simulink model "Mdl_Dim"  (R2024b)
settings: Solver=FixedStepDiscrete  StartTime=0.0  StopTime=10.0  FixedStep=0.1  RelTol=1e-3  EnableMultiTasking=on
values from neighbouring files (symbols this model uses):
  DEFAULT_MODE = mpt.Parameter    [Mdl_Dim_DD.m]
  DEFAULT_STEP = mpt.Parameter    [Mdl_Dim_DD.m]
  Mdl_Dim_cTaskPeriod = mpt.Parameter    [Mdl_Dim_rte_types.m]
  RTE_E_MAX_AGE_EXCEEDED = mpt.Parameter    [Mdl_Dim_rte_types.m]
  RTE_E_NEVER_RECEIVED = mpt.Parameter    [Mdl_Dim_rte_types.m]
  STATUS_OFF = mpt.Parameter    [Mdl_Dim_DD.m]
  STATUS_ON = mpt.Parameter    [Mdl_Dim_DD.m]
  SWITCHING_MECHANISM = mpt.Parameter    [Mdl_Dim_DD.m]
  ZERO_VAL = mpt.Parameter    [Mdl_Dim_DD.m]
undefined symbols (not defined in the file or in its folder): AppModule, CAN_COMUN_ACTIVE, CAN_COMUN_FAIL, CAN_VAL_OFF, CAN_VAL_ON, ChannelID, CLUSTER_ACTIVE, DAYNIGHT_STS_NOTRequire, DIAG_NCTRL, DIM_DAY_MODE, DIM_NIGHT_MODE, DOWN_THRESH_1SW, DrvRec_Rheo_down_Long_Press, DrvRec_Rheo_down_Short_Press, DrvRec_Rheo_up_Long_Press, DrvRec_Rheo_Up_Short_Press, DW_EVENT, DW_ON, eAppMdl_type_instance, eDayNightModeIn, eIllumination_levelIn, eSIGNAL_MISSING, eSIGNAL_NEVER_RECEIVED, eSleepSt_type_instance, FALSE, GetPwmDirect, GetPwmWithTime, GetPwmWithTimeExp, IgnOn, INDEX_MCUID0340, INDEX_MCUID0341, INDEX_MCUID0430, IoHwAb_PwmSignalIdType_type_instance, l_Wheel_Down_ParamArray, l_Wheel_Up_ParamArray, MAX_UINT16, MAXHOLD, MINHOLD, NETWORK_NORMAL, NETWORK_SLEEP, NETWORK_STANDALONE, NONE, NVM_Adapter_SetNVM_RheostatDayStep, NVM_Adapter_SetNVM_RheostatDayStepU1, NVM_Adapter_SetNVM_RheostatDayStepU2, NVM_Adapter_SetNVM_RheostatDayStepU3, NVM_Adapter_SetNVM_RheostatNightStep, NVM_Adapter_SetNVM_RheostatNightStepU1, NVM_Adapter_SetNVM_RheostatNightStepU2, NVM_Adapter_SetNVM_RheostatNightStepU3, OpeModeRheostatChange, pJustRcvdStatus, pNvmData, POS_MAX, POS_MIN, RHEO_1SW_TYPE, RHEO_2SW_TYPE, RHEO_SOFTSW_TYPE, RHEO_VALUE_FIVE_U16, RHEO_VALUE_ONE_BOOL ... (+48)
libraries: simulink x65
(part 2 of 4)

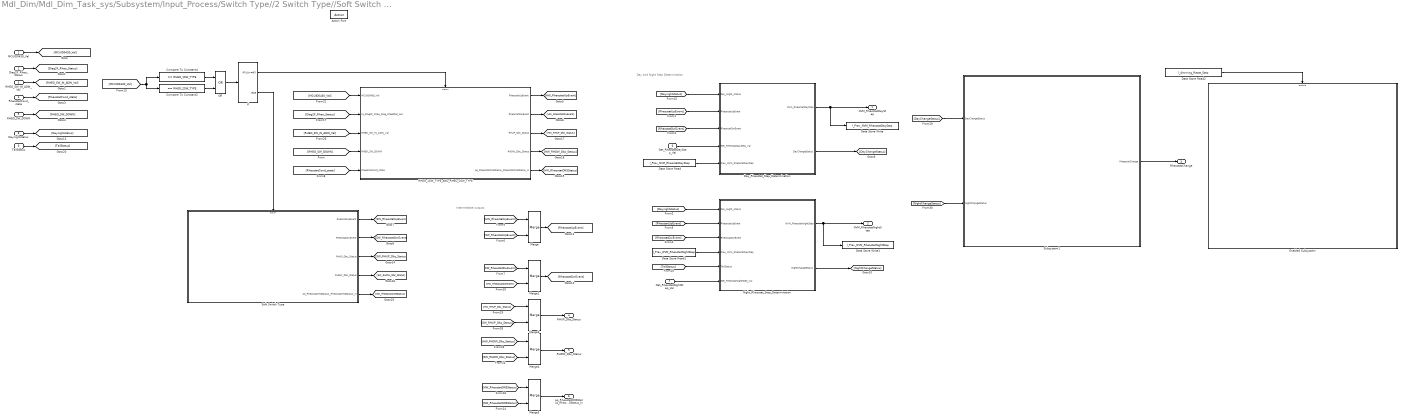
== system Mdl_Dim/Mdl_Dim_Task_sys/Subsystem/Input_Process/Switch Type//2 Switch Type//Soft Switch Type ==
  note: Intermediate outputs
  note: Day and Night Step Determination
  MCUID0430_Val : Inport
  Diag2F_Rheo_Status : Inport  Port=2
  RHEO_SW_IN_ADIN_Val : Inport  Port=3
  RheostatCond_state : Inport  Port=4
  RHEO_SW_DOWN : Inport  Port=5
  Get_RheostatDayStep_Val : Inport  Port=6
  Get_RheostatNightStep_Val : Inport  Port=7
  Daynightstatus : Inport  Port=8
  TailStatus : Inport  Port=9
  Action Port : ActionPort
  Compare To Constant2 : simulink/Logic and Bit Operations/Compare To Constant  relop===  const=RHEO_2SW_TYPE  OutDataTypeStr=boolean
  Compare To Constant4 : simulink/Logic and Bit Operations/Compare To Constant  relop===  const=RHEO_1SW_TYPE  OutDataTypeStr=boolean
  Data Store Read : DataStoreRead  DataStoreName=l_Prev_NVM_RheostatDayStep  IndexOptions=Index vector (dialog)  Indices=1  OutputSizes=1
  Data Store Read1 : DataStoreRead  DataStoreName=l_Prev_NVM_RheostatNightStep  IndexOptions=Index vector (dialog)  Indices=1  OutputSizes=1
  Data Store Read2 : DataStoreRead  DataStoreName=l_dimming_Reset_Step  IndexOptions=Index vector (dialog)  Indices=1  OutputSizes=1
  Data Store Write : DataStoreWrite  DataStoreName=l_Prev_NVM_RheostatDayStep  IndexOptions=Index vector (dialog)  Indices=1  OutputSizes=1
  Data Store Write1 : DataStoreWrite  DataStoreName=l_Prev_NVM_RheostatNightStep  IndexOptions=Index vector (dialog)  Indices=1  OutputSizes=1
  Day_Rheostat_Step_Determination : Truth Table  Priority=2  TreatAsAtomicUnit=on
      settings: RTWSystemCode=Nonreusable function  RTWFcnNameOpts=Use subsystem name
  Enabled Subsystem : Subsystem  Priority=3  TreatAsAtomicUnit=on
  If : If  IfExpression=(u1~=0)
  Merge{,1,3..5} (5 alike) : Merge
  Night_Rheostat_Step_Determination : Truth Table  Priority=2  TreatAsAtomicUnit=on
      settings: RTWSystemCode=Nonreusable function  RTWFcnNameOpts=Use subsystem name
  OR : Logic  Operator=OR  AllPortsSameDT=off  OutDataTypeStr=boolean
  RHEO_1SW_TYPE_AND_RHEO_2SW_TYPE : Subsystem  RTWFcnName=ONE_TWO_SWITCH_HANDLING
      settings: RTWSystemCode=Nonreusable function  RTWFcnNameOpts=User specified
  Soft Switch Type : Subsystem  RTWFcnName=SOFT_SWITCH_HANDLING
      settings: RTWSystemCode=Nonreusable function  RTWFcnNameOpts=User specified
  Subsystem1 : Subsystem  Priority=2
  "NVM_RheostatDayStep " : Outport  VectorParamsAs1DForOutWhenUnconnected=off
  NVM_RheostatNightStep : Outport  Port=2  VectorParamsAs1DForOutWhenUnconnected=off
  RheostatChange : Outport  Port=3  VectorParamsAs1DForOutWhenUnconnected=off
  RHUP_Dbc_Status : Outport  Port=4  VectorParamsAs1DForOutWhenUnconnected=off
  RHDW_Dbc_Status : Outport  Port=5  VectorParamsAs1DForOutWhenUnconnected=off
  pp_RheostatONSStatus_RheostatONSStatus_In : Outport  Port=6  VectorParamsAs1DForOutWhenUnconnected=off
  wires:
  [MCUID0430_Val] -> Compare To Constant4/1, Compare To Constant2/1
  [RheostatCond_state] -> RHEO_1SW_TYPE_AND_RHEO_2SW_TYPE/5(RheostatCond_state)
  [RHEO_SW_IN_ADIN_Val] -> RHEO_1SW_TYPE_AND_RHEO_2SW_TYPE/3(RHEO_SW_IN_ADIN_Val)
  [Diag2F_Rheo_Status] -> RHEO_1SW_TYPE_AND_RHEO_2SW_TYPE/2(rp_Diag2F_Rheo_Diag_RheoStat_out)
  [MCUID0430_Val] -> RHEO_1SW_TYPE_AND_RHEO_2SW_TYPE/1(MCUID0430_Val)
  Compare To Constant4/1 -> OR/1
  Compare To Constant2/1 -> OR/2
  MCUID0430_Val/1 -> [MCUID0430_Val]
  Diag2F_Rheo_Status/1 -> [Diag2F_Rheo_Status]
  RHEO_SW_IN_ADIN_Val/1 -> [RHEO_SW_IN_ADIN_Val]
  RheostatCond_state/1 -> [RheostatCond_state]
  RHEO_SW_DOWN/1 -> [RHEO_SW_DOWN]
  [RHEO_SW_DOWN] -> RHEO_1SW_TYPE_AND_RHEO_2SW_TYPE/4(RHEO_SW_DOWN)
  OR/1 -> If/1
  If/1 -> RHEO_1SW_TYPE_AND_RHEO_2SW_TYPE/Action
  If/2 -> Soft Switch Type/Action
  RHEO_1SW_TYPE_AND_RHEO_2SW_TYPE/1(RheostatUpEvent) -> [HW_RheostatUpEvent]
  RHEO_1SW_TYPE_AND_RHEO_2SW_TYPE/2(RheostatDwEvent) -> [HW_RheostatDwEvent]
  Soft Switch Type/1(RheostatUpEvent) -> [SW_RheostatUpEvent]
  Soft Switch Type/2(RheostatDwEvent) -> [SW_RheostatDwEvent]
  [HW_RheostatUpEvent] -> Merge/1
  [SW_RheostatUpEvent] -> Merge/2
  [SW_RheostatDwEvent] -> Merge1/1
  [HW_RheostatDwEvent] -> Merge1/2
  Merge/1 -> [RheostatUpEvent]
  Merge1/1 -> [RheostatDwEvent]
  [RheostatUpEvent] -> Day_Rheostat_Step_Determination/2(RheostatUpEvent)
  [RheostatDwEvent] -> Day_Rheostat_Step_Determination/3(RheostatDwEvent)
  Get_RheostatDayStep_Val/1 -> Day_Rheostat_Step_Determination/4(Get_RheostatDayStep_Val)
  [Daynightstatus] -> Day_Rheostat_Step_Determination/1(Day_Night_status)
  Day_Rheostat_Step_Determination/2(DayChangeStatus) -> [DayChangeStatus]
  Day_Rheostat_Step_Determination/1(NVM_RheostatDayStep) -> Data Store Write/1, "NVM_RheostatDayStep "/1
  Data Store Read/1 -> Day_Rheostat_Step_Determination/5(Prev_NVM_RheostatDayStep)
  Data Store Read1/1 -> Night_Rheostat_Step_Determination/4(Prev_NVM_RheostatDayStep)
  [TailStatus] -> Night_Rheostat_Step_Determination/5(TailStatus)
  [Daynightstatus] -> Night_Rheostat_Step_Determination/1(Day_Night_status)
  Night_Rheostat_Step_Determination/2(NightChangeStatus) -> [NightChangeStatus]
  [RheostatDwEvent] -> Night_Rheostat_Step_Determination/3(RheostatDwEvent)
  [RheostatUpEvent] -> Night_Rheostat_Step_Determination/2(RheostatUpEvent)
  Night_Rheostat_Step_Determination/1(NVM_RheostatNightStep) -> Data Store Write1/1, NVM_RheostatNightStep/1
  Get_RheostatNightStep_Val/1 -> Night_Rheostat_Step_Determination/6(Get_RheostatNightStep_Val)
  Daynightstatus/1 -> [Daynightstatus]
  Merge5/1 -> pp_RheostatONSStatus_RheostatONSStatus_In/1
  Soft Switch Type/3(RHUP_Dbc_Status) -> [SW_RHUP_Dbc_Status]
  Soft Switch Type/4(RHDW_Dbc_Status) -> [SW_RHDW_Dbc_Status]
  RHEO_1SW_TYPE_AND_RHEO_2SW_TYPE/3(RHUP_Dbc_Status) -> [HW_RHUP_Dbc_Status]
  RHEO_1SW_TYPE_AND_RHEO_2SW_TYPE/4(RHDW_Dbc_Status) -> [HW_RHDW_Dbc_Status]
  [HW_RHUP_Dbc_Status] -> Merge3/1
  [SW_RHUP_Dbc_Status] -> Merge3/2
  Merge3/1 -> RHUP_Dbc_Status/1
  [HW_RHDW_Dbc_Status] -> Merge4/1
  [SW_RHDW_Dbc_Status] -> Merge4/2
  Merge4/1 -> RHDW_Dbc_Status/1
  RHEO_1SW_TYPE_AND_RHEO_2SW_TYPE/5(pp_RheostatONSStatus_RheostatONSStatus_In) -> [HW_RheostatONSStatus]
  [SW_RheostatONSStatus] -> Merge5/2
  [HW_RheostatONSStatus] -> Merge5/1
  Soft Switch Type/5(pp_RheostatONSStatus_RheostatONSStatus_In) -> [SW_RheostatONSStatus]
  TailStatus/1 -> [TailStatus]
  Subsystem1/1(RheostatChange) -> RheostatChange/1
  [NightChangeStatus] -> Subsystem1/2(NightChangeStatus)
  [DayChangeStatus] -> Subsystem1/1(DayChangeStatus)
  Data Store Read2/1 -> Enabled Subsystem/Enable

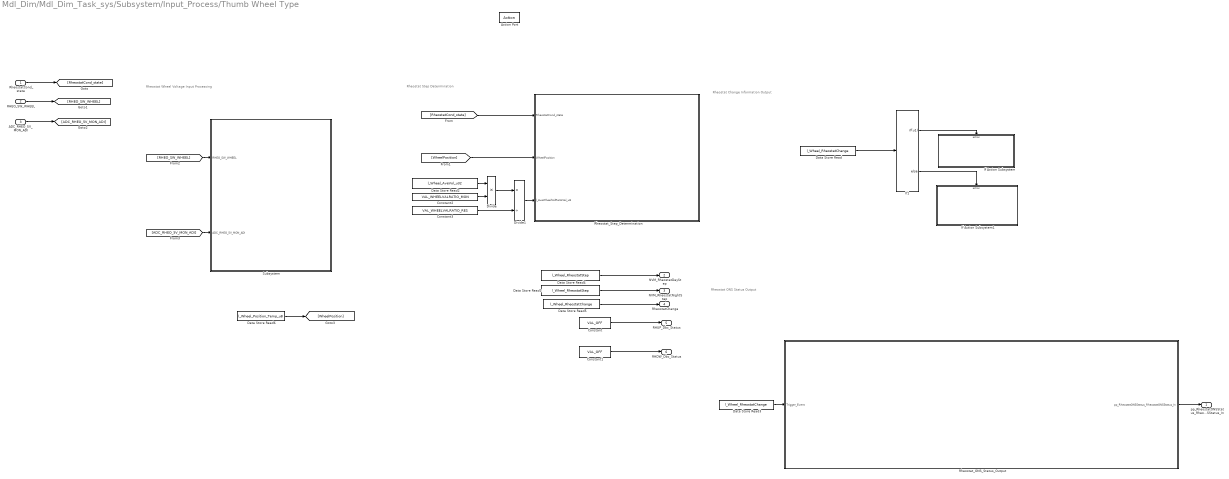
== system Mdl_Dim/Mdl_Dim_Task_sys/Subsystem/Input_Process/Thumb Wheel Type ==
  note: Rheostat Wheel Voltage Input Processing
  note: Rheostat Step Determination
  note: Rheostat Change Information Output
  note: Rheostat ONS Status Output
  RheostatCond_state : Inport
  RHEO_SW_WHEEL : Inport  Port=2
  ADC_RHEO_5V_MON_ADI : Inport  Port=3
  Action Port : ActionPort
  Constant : Constant  Value=VAL_OFF
  Constant1 : Constant  Value=VAL_OFF
  Constant2 : Constant  Value=VAL_WHEELVALRATIO_MON
  Constant3 : Constant  Value=VAL_WHEELVALRATIO_RES
  Data Store Read : DataStoreRead  DataStoreName=l_Wheel_RheostatChange  IndexOptions=Index vector (dialog)  Indices=1  OutputSizes=1
  Data Store Read1 : DataStoreRead  DataStoreName=l_Wheel_RheostatStep  IndexOptions=Index vector (dialog)  Indices=1  OutputSizes=1
  Data Store Read2 : DataStoreRead  DataStoreName=l_Wheel_AveVol_u32  IndexOptions=Index vector (dialog)  Indices=1  OutputSizes=1
  Data Store Read3 : DataStoreRead  DataStoreName=l_Wheel_RheostatChange  IndexOptions=Index vector (dialog)  Indices=1  OutputSizes=1
  Data Store Read4 : DataStoreRead  DataStoreName=l_Wheel_RheostatStep  IndexOptions=Index vector (dialog)  Indices=1  OutputSizes=1
  Data Store Read5 : DataStoreRead  DataStoreName=l_Wheel_RheostatChange  IndexOptions=Index vector (dialog)  Indices=1  OutputSizes=1
  Data Store Read6 : DataStoreRead  DataStoreName=l_Wheel_Position_Temp_u8  IndexOptions=Index vector (dialog)  Indices=1  OutputSizes=1
  Divide : Product  OutDataTypeStr=uint32
  Divide1 : Product  Inputs=*/  OutDataTypeStr=uint8
  If Action Subsystem : Subsystem  TreatAsAtomicUnit=on
  If Action Subsystem1 : Subsystem  TreatAsAtomicUnit=on
  If1 : If  IfExpression=u1
  "Rheostat_ONS_Status_Output " : Subsystem
  Rheostat_Step_Determination : Truth Table  TreatAsAtomicUnit=on
      settings: RTWSystemCode=Nonreusable function  RTWFcnNameOpts=Use subsystem name
  Subsystem : Subsystem
  pp_RheostatONSStatus_RheostatONSStatus_In : Outport  VectorParamsAs1DForOutWhenUnconnected=off
  "NVM_RheostatDayStep " : Outport  Port=2  VectorParamsAs1DForOutWhenUnconnected=off
  NVM_RheostatNightStep : Outport  Port=3  VectorParamsAs1DForOutWhenUnconnected=off
  RheostatChange : Outport  Port=4  VectorParamsAs1DForOutWhenUnconnected=off
  RHUP_Dbc_Status : Outport  Port=5  VectorParamsAs1DForOutWhenUnconnected=off
  RHDW_Dbc_Status : Outport  Port=6  VectorParamsAs1DForOutWhenUnconnected=off
  wires:
  "Rheostat_ONS_Status_Output "/1(pp_RheostatONSStatus_RheostatONSStatus_In) -> pp_RheostatONSStatus_RheostatONSStatus_In/1
  If1/2 -> If Action Subsystem1/Action
  If1/1 -> If Action Subsystem/Action
  Data Store Read/1 -> If1/1
  RHEO_SW_WHEEL/1 -> [RHEO_SW_WHEEL]
  ADC_RHEO_5V_MON_ADI/1 -> [ADC_RHEO_5V_MON_ADI]
  RheostatCond_state/1 -> [RheostatCond_state]
  [RheostatCond_state] -> Rheostat_Step_Determination/1(RheostatCond_state)
  Data Store Read5/1 -> RheostatChange/1
  Constant/1 -> RHUP_Dbc_Status/1
  Constant1/1 -> RHDW_Dbc_Status/1
  [WheelPosition] -> Rheostat_Step_Determination/2(WheelPosition)
  [RHEO_SW_WHEEL] -> Subsystem/1(RHEO_SW_WHEEL)
  [ADC_RHEO_5V_MON_ADI] -> Subsystem/2(ADC_RHEO_5V_MON_ADI)
  Data Store Read6/1 -> [WheelPosition]
  Data Store Read3/1 -> "Rheostat_ONS_Status_Output "/1(Trigger_Event)
  Data Store Read4/1 -> "NVM_RheostatDayStep "/1
  Data Store Read1/1 -> NVM_RheostatNightStep/1
  Constant3/1 -> Divide1/2
  Divide/1 -> Divide1/1
  Data Store Read2/1 -> Divide/1
  Constant2/1 -> Divide/2
  Divide1/1 -> Rheostat_Step_Determination/3(l_AveWheelVolRaitoVal_u8)

== system Mdl_Dim/Mdl_Dim_Task_sys/Subsystem/Input_Process/Switch Type//2 Switch Type//Soft Switch Type/Enabled Subsystem ==
  Enable : EnablePort
  Constant : Constant  Value=VAL_OFF
  Constant1 : Constant  Value=MAXHOLD
  Data Store Read : DataStoreRead  DataStoreName=l_Dim_MCUID0340_val  IndexOptions=Index vector (dialog)  Indices=1  OutputSizes=1
  Data Store Write : DataStoreWrite  DataStoreName=l_Prev_NVM_RheostatDayStep  IndexOptions=Index vector (dialog)  Indices=1  OutputSizes=1
  Data Store Write1 : DataStoreWrite  DataStoreName=l_Prev_NVM_RheostatNightStep  IndexOptions=Index vector (dialog)  Indices=1  OutputSizes=1
  Data Store Write2 : DataStoreWrite  DataStoreName=l_dimming_Reset_Step  IndexOptions=Index vector (dialog)  Indices=1  OutputSizes=1
  NVM_Adapter_SetNVM_RheostatDayStep : FunctionCaller  FunctionPrototype=NVM_Adapter_SetNVM_RheostatDayStep(pNvmData)  InputArgumentSpecifications=uint8(1)  OutputArgumentSpecifications=<Enter example>
  NVM_Adapter_SetNVM_RheostatDayStepU1 : FunctionCaller  FunctionPrototype=NVM_Adapter_SetNVM_RheostatDayStepU1(pNvmData)  InputArgumentSpecifications=uint8(1)  OutputArgumentSpecifications=<Enter example>
  NVM_Adapter_SetNVM_RheostatDayStepU2 : FunctionCaller  FunctionPrototype=NVM_Adapter_SetNVM_RheostatDayStepU2(pNvmData)  InputArgumentSpecifications=uint8(1)  OutputArgumentSpecifications=<Enter example>
  NVM_Adapter_SetNVM_RheostatDayStepU3 : FunctionCaller  FunctionPrototype=NVM_Adapter_SetNVM_RheostatDayStepU3(pNvmData)  InputArgumentSpecifications=uint8(1)  OutputArgumentSpecifications=<Enter example>
  NVM_Adapter_SetNVM_RheostatNightStep : FunctionCaller  FunctionPrototype=NVM_Adapter_SetNVM_RheostatNightStep(pNvmData)  InputArgumentSpecifications=uint8(1)  OutputArgumentSpecifications=<Enter example>
  NVM_Adapter_SetNVM_RheostatNightStep2 : FunctionCaller  FunctionPrototype=NVM_Adapter_SetNVM_RheostatNightStepU2(pNvmData)  InputArgumentSpecifications=uint8(1)  OutputArgumentSpecifications=<Enter example>
  NVM_Adapter_SetNVM_RheostatNightStepU1 : FunctionCaller  FunctionPrototype=NVM_Adapter_SetNVM_RheostatNightStepU1(pNvmData)  InputArgumentSpecifications=uint8(1)  OutputArgumentSpecifications=<Enter example>
  NVM_Adapter_SetNVM_RheostatNightStepU3 : FunctionCaller  FunctionPrototype=NVM_Adapter_SetNVM_RheostatNightStepU3(pNvmData)  InputArgumentSpecifications=uint8(1)  OutputArgumentSpecifications=<Enter example>
  wires:
  Constant/1 -> Data Store Write2/1
  Constant1/1 -> Data Store Write/1, NVM_Adapter_SetNVM_RheostatDayStep/1, NVM_Adapter_SetNVM_RheostatDayStepU3/1, NVM_Adapter_SetNVM_RheostatDayStepU2/1, NVM_Adapter_SetNVM_RheostatDayStepU1/1
  Data Store Read/1 -> NVM_Adapter_SetNVM_RheostatNightStep2/1, Data Store Write1/1, NVM_Adapter_SetNVM_RheostatNightStep/1, NVM_Adapter_SetNVM_RheostatNightStepU3/1, NVM_Adapter_SetNVM_RheostatNightStepU1/1

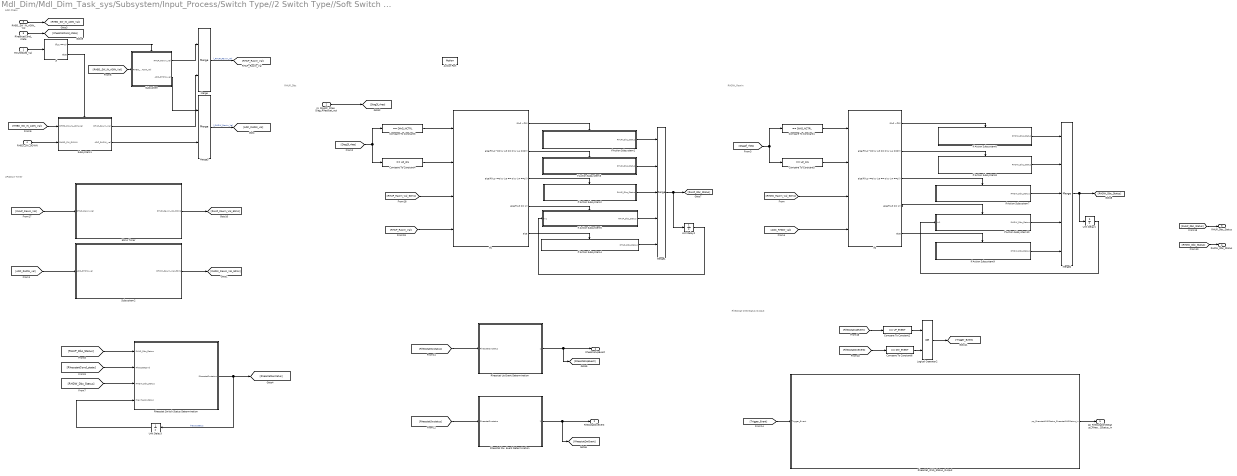
== system Mdl_Dim/Mdl_Dim_Task_sys/Subsystem/Input_Process/Switch Type//2 Switch Type//Soft Switch Type/RHEO_1SW_TYPE_AND_RHEO_2SW_TYPE ==
  note: Rheostat ONS Status Output
  note: RHDW_RawIn
  note: RHUP_Dbc
  note: UP/Down Timer
  note: ADC Check
  MCUID0430_Val : Inport
  rp_Diag2F_Rheo_Diag_RheoStat_out : Inport  Port=2
  RHEO_SW_IN_ADIN_Val : Inport  Port=3
  RHEO_SW_DOWN : Inport  Port=4
  RheostatCond_state : Inport  Port=5
  Action Port : ActionPort
  " Rheostat Dw  Event Determination" : Subsystem
  " Rheostat Up Event Determination" : Subsystem
  50ms Timer : Subsystem  Priority=1
      settings: AttributesFormatString=Priority = %<Priority>
  Compare To Constant1 : simulink/Logic and Bit Operations/Compare To Constant  relop===  const=DIAG_NCTRL  OutDataTypeStr=boolean
  Compare To Constant2 : simulink/Logic and Bit Operations/Compare To Constant  relop===  const=UP_EVENT  OutDataTypeStr=boolean
  Compare To Constant3 : simulink/Logic and Bit Operations/Compare To Constant  relop===  const=DIAG_NCTRL  OutDataTypeStr=boolean
  Compare To Constant4 : simulink/Logic and Bit Operations/Compare To Constant  relop===  const=UP_ON  OutDataTypeStr=boolean
  Compare To Constant5 : simulink/Logic and Bit Operations/Compare To Constant  relop===  const=UP_ON  OutDataTypeStr=boolean
  Compare To Constant6 : simulink/Logic and Bit Operations/Compare To Constant  relop===  const=DW_EVENT  OutDataTypeStr=boolean
  If : If  IfExpression=u1 == 0
  If Action Subsystem1 : Subsystem  TreatAsAtomicUnit=on
  If Action Subsystem10 : Subsystem  TreatAsAtomicUnit=on
  If Action Subsystem2 : Subsystem  TreatAsAtomicUnit=on
  If Action Subsystem3 : Subsystem  TreatAsAtomicUnit=on
  If Action Subsystem4 : Subsystem  TreatAsAtomicUnit=on
  If Action Subsystem5 : Subsystem  TreatAsAtomicUnit=on
  If Action Subsystem6 : Subsystem  TreatAsAtomicUnit=on
  If Action Subsystem7 : Subsystem  TreatAsAtomicUnit=on
  If Action Subsystem8 : Subsystem  TreatAsAtomicUnit=on
  If Action Subsystem9 : Subsystem  TreatAsAtomicUnit=on
  If1 : If  Priority=3  NumInputs=4  IfExpression=u2 ~=0  ElseIfExpressions=((u1~=0) & (u3 == 0) & (u4 ==0)) , ((u1~=0) & (u3 == 0) & (u4 ==1)),(u3 == 1)
      settings: AttributesFormatString=Priority = %<Priority>
  If2 : If  NumInputs=4  IfExpression=u2 ~=0  ElseIfExpressions=((u1~=0) & (u3 == 0) & (u4 ==0)) , ((u1~=0) & (u3 == 0) & (u4 ==1)),(u3 == 1)
  Logical Operator2 : Logic  Operator=OR  AllPortsSameDT=off  OutDataTypeStr=boolean
  Merge : Merge
  Merge1 : Merge  Inputs=5
  Merge2 : Merge  Inputs=5
  Merge3 : Merge
  Rheostat Switch Status Determination : Truth Table
  "Rheostat_ONS_Status_Output " : Subsystem
  Subsystem : Subsystem
  Subsystem1 : Subsystem
  Subsystem2 : Subsystem  Priority=2
      settings: AttributesFormatString=Priority = %<Priority>
  Unit Delay1 : UnitDelay  SampleTime=-1  StateName=l_Prev_SW1RHDW_Dbc_status  HasFrameUpgradeWarning=on
  Unit Delay2 : UnitDelay  SampleTime=-1  StateName=l_Prev_SW1RHUP_Dbc_status  HasFrameUpgradeWarning=on
  Unit Delay3 : UnitDelay  InitialCondition=UNKNOWNSTATUS  SampleTime=-1  StateName=l_Prev_RheostatswStatus  HasFrameUpgradeWarning=on
  RheostatUpEvent : Outport  VectorParamsAs1DForOutWhenUnconnected=off
  RheostatDwEvent : Outport  Port=2  VectorParamsAs1DForOutWhenUnconnected=off
  RHUP_Dbc_Status : Outport  Port=3  VectorParamsAs1DForOutWhenUnconnected=off
  RHDW_Dbc_Status : Outport  Port=4  VectorParamsAs1DForOutWhenUnconnected=off
  pp_RheostatONSStatus_RheostatONSStatus_In : Outport  Port=5  VectorParamsAs1DForOutWhenUnconnected=off
  wires:
  If1/3 -> If Action Subsystem2/Action
  Merge1/1 -> [RHUP_Dbc_Status], Unit Delay2/1
  Unit Delay2/1 -> If Action Subsystem5/1(In1)
  50ms Timer/1(RHUP_RawIn_Val_50ms) -> [RHUP_RawIn_Val_50ms]
  If Action Subsystem5/1(RHUP_Dbc_Status) -> Merge1/4
  Compare To Constant3/1 -> If1/1
  If1/2 -> If Action Subsystem3/Action
  If Action Subsystem4/1(RHUP_Dbc_Status) -> Merge1/5
  If1/4 -> If Action Subsystem5/Action
  [RHUP_RawIn_Val] -> If1/4
  If1/5 -> If Action Subsystem4/Action
  If Action Subsystem2/1(RHUP_Dbc_Status) -> Merge1/3
  If Action Subsystem1/1(RHUP_Dbc_Status) -> Merge1/1
  Compare To Constant4/1 -> If1/2
  [RHUP_RawIn_Val_50ms] -> If1/3
  [RHUP_RawIn_Val] -> 50ms Timer/1(RHUP_RawIn_Val)
  If1/1 -> If Action Subsystem1/Action
  If Action Subsystem3/1(RHUP_Dbc_Status) -> Merge1/2
  [Diag2f_rheo] -> Compare To Constant1/1, Compare To Constant5/1
  If2/1 -> If Action Subsystem6/Action
  If Action Subsystem8/1(RHDW_Dbc_Status) -> Merge2/2
  If Action Subsystem6/1(RHDW_Dbc_Status) -> Merge2/1
  If Action Subsystem7/1(RHDW_Dbc_Status) -> Merge2/3
  [RHDW_RawIn_Val_50ms] -> If2/3
  Compare To Constant5/1 -> If2/2
  [ADC_RHDW_val] -> If2/4
  If2/5 -> If Action Subsystem9/Action
  If2/4 -> If Action Subsystem10/Action
  If Action Subsystem9/1(RHDW_Dbc_Status) -> Merge2/5
  If2/2 -> If Action Subsystem8/Action
  Compare To Constant1/1 -> If2/1
  Merge2/1 -> Unit Delay1/1, [RHDW_Dbc_Status]
  Unit Delay1/1 -> If Action Subsystem10/1(In1)
  If Action Subsystem10/1(RHDW_Dbc_Status) -> Merge2/4
  If2/3 -> If Action Subsystem7/Action
  Subsystem2/1(RHDW_RawIn_Val_50ms) -> [RHDW_RawIn_Val_50ms]
  [ADC_RHDW_val] -> Subsystem2/1(ADC_RHDW_val)
  rp_Diag2F_Rheo_Diag_RheoStat_out/1 -> [Diag2f_rheo]
  [Diag2f_rheo] -> Compare To Constant4/1, Compare To Constant3/1
  RHEO_SW_IN_ADIN_Val/1 -> [RHEO_SW_IN_ADIN_Val]
  [RHEO_SW_IN_ADIN_Val] -> Subsystem/1(RHEO_SW_IN_ADIN_Val)
  RHEO_SW_DOWN/1 -> Subsystem1/2(RHEO_SW_DOWN)
  [RHEO_SW_IN_ADIN_Val] -> Subsystem1/1(RHEO_SW_IN_ADIN_Val)
  MCUID0430_Val/1 -> If/1
  If/1 -> Subsystem/Action
  If/2 -> Subsystem1/Action
  Subsystem/1(RHUP_RawIn_Val) -> Merge/1
  Subsystem1/1(RHUP_RawIn_Val) -> Merge/2
  Subsystem/2(ADC_RHDW_val) -> Merge3/1
  Subsystem1/2(ADC_RHDW_val) -> Merge3/2
  Merge/1 -> [RHUP_RawIn_Val]  "l_RHUP_RawIn_Val"
  Merge3/1 -> [ADC_RHDW_val]  "l_RHDW_RawIn_Val"
  [RheostatCond_state] -> Rheostat Switch Status Determination/2(RheostatCond)
  [RHUP_Dbc_Status] -> Rheostat Switch Status Determination/1(RHUP_Dbc_Status)
  Unit Delay3/1 -> Rheostat Switch Status Determination/4(Prevrheoswstatus)
  Rheostat Switch Status Determination/1(RheostatSwstatus) -> Unit Delay3/1, [RheostatSwstatus]  "rheoswstatus"
  [RHDW_Dbc_Status] -> Rheostat Switch Status Determination/3(RHDW_Dbc_Status)
  [RheostatSwstatus] -> " Rheostat Dw  Event Determination"/1(RheostatSwstatus)
  " Rheostat Dw  Event Determination"/1(" ") -> [RheostatDwEvent], RheostatDwEvent/1
  [RheostatSwstatus] -> " Rheostat Up Event Determination"/1(RheostatSwstatus)
  " Rheostat Up Event Determination"/1(" ") -> [RheostatUpEvent], RheostatUpEvent/1
  RheostatCond_state/1 -> [RheostatCond_state]
  [RHDW_Dbc_Status] -> RHDW_Dbc_Status/1
  [RHUP_Dbc_Status] -> RHUP_Dbc_Status/1
  [RheostatUpEvent] -> Compare To Constant2/1
  [RheostatDwEvent] -> Compare To Constant6/1
  Compare To Constant2/1 -> Logical Operator2/1
  Compare To Constant6/1 -> Logical Operator2/2
  Logical Operator2/1 -> [Trigger_Event]
  "Rheostat_ONS_Status_Output "/1(pp_RheostatONSStatus_RheostatONSStatus_In) -> pp_RheostatONSStatus_RheostatONSStatus_In/1
  [Trigger_Event] -> "Rheostat_ONS_Status_Output "/1(Trigger_Event)

== system Mdl_Dim/Mdl_Dim_Task_sys/Subsystem/Input_Process/Switch Type//2 Switch Type//Soft Switch Type/Soft Switch Type ==
  Action Port : ActionPort
  Constant : Constant  Value=VAL_OFF
  Constant1 : Constant  Value=VAL_OFF
  Constant2 : Constant  Value=VAL_OFF
  Constant3 : Constant  Value=VAL_OFF  OutDataTypeStr=uint32
  Data Store Write : DataStoreWrite  DataStoreName=l_Prev_Rheo3secCount  IndexOptions=Index vector (dialog)  Indices=1  OutputSizes=1
  Event Check : Subsystem  Priority=1
      settings: AttributesFormatString=Priority = %<Priority>
  Event Clear : Subsystem  Priority=2
      settings: AttributesFormatString=Priority = %<Priority>
  RheostatUpEvent : Outport  VectorParamsAs1DForOutWhenUnconnected=off
  RheostatDwEvent : Outport  Port=2  VectorParamsAs1DForOutWhenUnconnected=off
  RHUP_Dbc_Status : Outport  Port=3  VectorParamsAs1DForOutWhenUnconnected=off
  RHDW_Dbc_Status : Outport  Port=4  VectorParamsAs1DForOutWhenUnconnected=off
  pp_RheostatONSStatus_RheostatONSStatus_In : Outport  Port=5  VectorParamsAs1DForOutWhenUnconnected=off
  wires:
  Event Check/1(RheostatUpEvent) -> RheostatUpEvent/1
  Event Check/2(RheostatDwEvent) -> RheostatDwEvent/1
  Constant/1 -> RHUP_Dbc_Status/1
  Constant1/1 -> RHDW_Dbc_Status/1
  Constant2/1 -> pp_RheostatONSStatus_RheostatONSStatus_In/1
  Constant3/1 -> Data Store Write/1

== system Mdl_Dim/Mdl_Dim_Task_sys/Subsystem/Input_Process/Switch Type//2 Switch Type//Soft Switch Type/Subsystem1 ==
  note: Change Judgement
  DayChangeStatus : Inport
  NightChangeStatus : Inport  Port=2
  If Action Subsystem : Subsystem  TreatAsAtomicUnit=on
  If Action Subsystem1 : Subsystem  TreatAsAtomicUnit=on
  If1 : If  IfExpression=u1
  Logical Operator : Logic  Operator=OR  AllPortsSameDT=off  OutDataTypeStr=boolean
  Merge2 : Merge
  RheostatChange : Outport  VectorParamsAs1DForOutWhenUnconnected=off
  wires:
  If1/1 -> If Action Subsystem/Action
  Logical Operator/1 -> If1/1
  Merge2/1 -> RheostatChange/1
  If Action Subsystem1/1(RheostatChange) -> Merge2/2
  If1/2 -> If Action Subsystem1/Action
  [NightChangeStatus] -> Logical Operator/2
  If Action Subsystem/1(RheostatChange) -> Merge2/1
  [DayChangeStatus] -> Logical Operator/1
  DayChangeStatus/1 -> [DayChangeStatus]
  NightChangeStatus/1 -> [NightChangeStatus]

== system Mdl_Dim/Mdl_Dim_Task_sys/Subsystem/Input_Process/Thumb Wheel Type/If Action Subsystem ==
  Action Port : ActionPort
  Data Store Read1 : DataStoreRead  DataStoreName=l_Wheel_RheostatStep  IndexOptions=Index vector (dialog)  Indices=1  OutputSizes=1
  Data Store Read4 : DataStoreRead  DataStoreName=l_Wheel_RheostatStep  IndexOptions=Index vector (dialog)  Indices=1  OutputSizes=1
  NVM_Adapter_SetNVM_RheostatDayStep : FunctionCaller  FunctionPrototype=NVM_Adapter_SetNVM_RheostatDayStep(pNvmData)  InputArgumentSpecifications=uint8(1)  OutputArgumentSpecifications=<Enter example>
  NVM_Adapter_SetNVM_RheostatNightStep : FunctionCaller  FunctionPrototype=NVM_Adapter_SetNVM_RheostatNightStep(pNvmData)  InputArgumentSpecifications=uint8(1)  OutputArgumentSpecifications=<Enter example>
  OpeModeRheostatChange : FunctionCaller  FunctionPrototype=OpeModeRheostatChange()  InputArgumentSpecifications=<Enter example>  OutputArgumentSpecifications=<Enter example>
  wires:
  Data Store Read1/1 -> NVM_Adapter_SetNVM_RheostatNightStep/1
  Data Store Read4/1 -> NVM_Adapter_SetNVM_RheostatDayStep/1

== system Mdl_Dim/Mdl_Dim_Task_sys/Subsystem/Input_Process/Thumb Wheel Type/If Action Subsystem1 ==
  Action Port : ActionPort

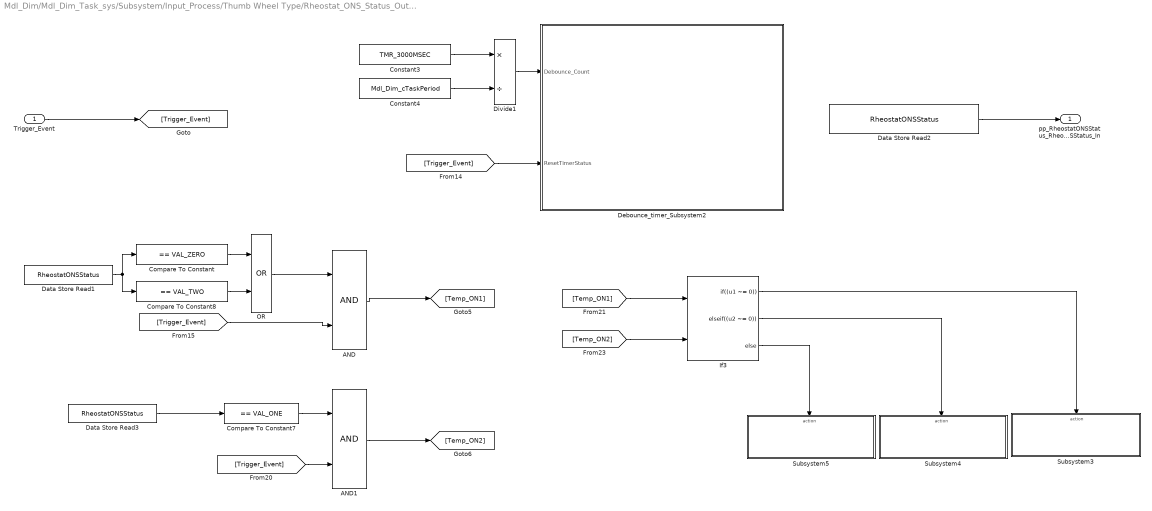
== system Mdl_Dim/Mdl_Dim_Task_sys/Subsystem/Input_Process/Thumb Wheel Type/Rheostat_ONS_Status_Output  ==
  Trigger_Event : Inport
  AND : Logic  AllPortsSameDT=off  OutDataTypeStr=boolean
  AND1 : Logic  AllPortsSameDT=off  OutDataTypeStr=boolean
  Compare To Constant : simulink/Logic and Bit Operations/Compare To Constant  relop===  const=VAL_ZERO  OutDataTypeStr=boolean
  Compare To Constant7 : simulink/Logic and Bit Operations/Compare To Constant  relop===  const=VAL_ONE  OutDataTypeStr=boolean
  Compare To Constant8 : simulink/Logic and Bit Operations/Compare To Constant  relop===  const=VAL_TWO  OutDataTypeStr=boolean
  Constant3 : Constant  Value=TMR_3000MSEC
  Constant4 : Constant  Value=Mdl_Dim_cTaskPeriod
  Data Store Read1 : DataStoreRead  DataStoreName=RheostatONSStatus  IndexOptions=Index vector (dialog)  Indices=1  OutputSizes=1
  Data Store Read2 : DataStoreRead  DataStoreName=RheostatONSStatus  IndexOptions=Index vector (dialog)  Indices=1  OutputSizes=1
  Data Store Read3 : DataStoreRead  DataStoreName=RheostatONSStatus  IndexOptions=Index vector (dialog)  Indices=1  OutputSizes=1
  Debounce_timer_Subsystem2 : Subsystem  Description=|
      | Input 1 : Deboune Count
      | Input 2 : Reset Timer Status
      | Output : Timer Debounce Status
  Divide1 : Product  Inputs=*/  OutDataTypeStr=uint16
  If3 : If  NumInputs=2  IfExpression=(u1 ~= 0)  ElseIfExpressions=(u2 ~= 0)
  OR : Logic  Operator=OR  AllPortsSameDT=off  OutDataTypeStr=boolean
  Subsystem3 : Subsystem
  Subsystem4 : Subsystem
  Subsystem5 : Subsystem
  pp_RheostatONSStatus_RheostatONSStatus_In : Outport  VectorParamsAs1DForOutWhenUnconnected=off
  wires:
  [Trigger_Event] -> AND1/2
  If3/3 -> Subsystem5/Action
  If3/2 -> Subsystem4/Action
  Constant3/1 -> Divide1/1
  Data Store Read1/1 -> Compare To Constant/1, Compare To Constant8/1
  Data Store Read3/1 -> Compare To Constant7/1
  [Temp_ON2] -> If3/2
  [Temp_ON1] -> If3/1
  AND1/1 -> [Temp_ON2]
  Data Store Read2/1 -> pp_RheostatONSStatus_RheostatONSStatus_In/1
  If3/1 -> Subsystem3/Action
  Compare To Constant/1 -> OR/1
  Compare To Constant7/1 -> AND1/1
  Compare To Constant8/1 -> OR/2
  Constant4/1 -> Divide1/2
  Divide1/1 -> Debounce_timer_Subsystem2/1(Debounce_Count)
  OR/1 -> AND/1
  [Trigger_Event] -> AND/2
  AND/1 -> [Temp_ON1]
  [Trigger_Event] -> Debounce_timer_Subsystem2/2("ResetTimerStatus ")
  Trigger_Event/1 -> [Trigger_Event]

== system Mdl_Dim/Mdl_Dim_Task_sys/Subsystem/Input_Process/Thumb Wheel Type/Subsystem ==
  RHEO_SW_WHEEL : Inport
  ADC_RHEO_5V_MON_ADI : Inport  Port=2
  Subsystem1 : Subsystem
  wires:
  RHEO_SW_WHEEL/1 -> [RHEO_SW_WHEEL]
  ADC_RHEO_5V_MON_ADI/1 -> [ADC_RHEO_5V_MON_ADI]
  [RHEO_SW_WHEEL] -> Subsystem1/1(RHEO_SW_WHEEL)
  [ADC_RHEO_5V_MON_ADI] -> Subsystem1/2(ADC_RHEO_5V_MON_ADI)

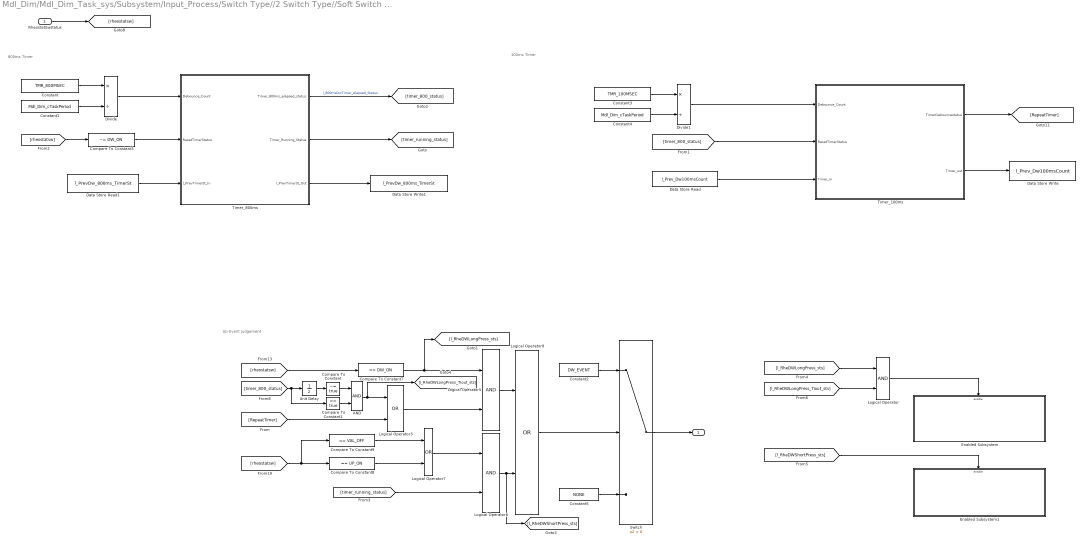
== system Mdl_Dim/Mdl_Dim_Task_sys/Subsystem/Input_Process/Switch Type//2 Switch Type//Soft Switch Type/RHEO_1SW_TYPE_AND_RHEO_2SW_TYPE/ Rheostat Dw  Event Determination ==
  note: 100ms Timer
  note: 800ms Timer
  note: Up Event judgement
  RheostatSwstatus : Inport
  AND : Logic  AllPortsSameDT=off  OutDataTypeStr=boolean
  Compare To Constant : simulink/Logic and Bit Operations/Compare To Constant  relop=~=  const=true  OutDataTypeStr=boolean
  Compare To Constant1 : simulink/Logic and Bit Operations/Compare To Constant  relop===  const=true  OutDataTypeStr=boolean
  Compare To Constant3 : simulink/Logic and Bit Operations/Compare To Constant  relop=~=  const=DW_ON  OutDataTypeStr=boolean
  Compare To Constant7 : simulink/Logic and Bit Operations/Compare To Constant  relop===  const=DW_ON  OutDataTypeStr=boolean
  Compare To Constant8 : simulink/Logic and Bit Operations/Compare To Constant  relop===  const=UP_ON  OutDataTypeStr=boolean
  Compare To Constant9 : simulink/Logic and Bit Operations/Compare To Constant  relop===  const=VAL_OFF  OutDataTypeStr=boolean
  Constant : Constant  Value=TMR_800MSEC
  Constant1 : Constant  Value=Mdl_Dim_cTaskPeriod
  Constant2 : Constant  Value=DW_EVENT
  Constant3 : Constant  Value=TMR_100MSEC
  Constant4 : Constant  Value=Mdl_Dim_cTaskPeriod
  Constant5 : Constant  Value=NONE
  Data Store Read : DataStoreRead  DataStoreName=l_Prev_Dw100msCount  IndexOptions=Index vector (dialog)  Indices=1  OutputSizes=1
  Data Store Read1 : DataStoreRead  DataStoreName=l_PrevDw_800ms_TimerSt  IndexOptions=Index vector (dialog)  Indices=1  OutputSizes=1
  Data Store Write : DataStoreWrite  DataStoreName=l_Prev_Dw100msCount  IndexOptions=Index vector (dialog)  Indices=1  OutputSizes=1
  Data Store Write1 : DataStoreWrite  DataStoreName=l_PrevDw_800ms_TimerSt  IndexOptions=Index vector (dialog)  Indices=1  OutputSizes=1
  Divide : Product  Inputs=*/  OutDataTypeStr=uint16
  Divide1 : Product  Inputs=*/  OutDataTypeStr=uint16
  Enabled Subsystem : Subsystem  TreatAsAtomicUnit=on
  Enabled Subsystem1 : Subsystem  TreatAsAtomicUnit=on
  Logical Operator : Logic  AllPortsSameDT=off  OutDataTypeStr=boolean
  Logical Operator3 : Logic  Operator=OR  AllPortsSameDT=off  OutDataTypeStr=boolean
  Logical Operator5 : Logic  AllPortsSameDT=off  OutDataTypeStr=boolean
  Logical Operator6 : Logic  AllPortsSameDT=off  OutDataTypeStr=boolean
  Logical Operator7 : Logic  Operator=OR  AllPortsSameDT=off  OutDataTypeStr=boolean
  Logical Operator8 : Logic  Operator=OR  AllPortsSameDT=off  OutDataTypeStr=boolean
  Switch : Switch  Criteria=u2 > Threshold  SaturateOnIntegerOverflow=off  InputSameDT=off
  Timer_100ms : Subsystem  Description=|  TreatAsAtomicUnit=on  RTWFcnName=Timer_100ms
      | Input 1 : Deboune Count
      | Input 2 : Reset Timer Status
      | Output : Timer Debounce Status
      settings: RTWFcnNameOpts=User specified
  Timer_800ms : Subsystem  Description=|  TreatAsAtomicUnit=on  RTWFcnName=Timer_800ms
      | Input 1 : Deboune Count
      | Input 2 : Reset Timer Status
      | Output : Timer Debounce Status
      settings: RTWFcnNameOpts=User specified
  Unit Delay : UnitDelay  SampleTime=-1  StateName=Prev_Dw_timer_800_status  HasFrameUpgradeWarning=on
  " " : Outport  VectorParamsAs1DForOutWhenUnconnected=off
  wires:
  Constant1/1 -> Divide/2
  Constant/1 -> Divide/1
  Timer_800ms/1(Timer_800ms_elapsed_status) -> [timer_800_status]  "l_800msDwTimer_elapsed_Status"
  Divide/1 -> Timer_800ms/1(Debounce_Count)
  Constant3/1 -> Divide1/1
  Constant4/1 -> Divide1/2
  RheostatSwstatus/1 -> [rheostatsw]
  [rheostatsw] -> Compare To Constant3/1
  Compare To Constant3/1 -> Timer_800ms/2("ResetTimerStatus ")
  Divide1/1 -> Timer_100ms/1(Debounce_Count)
  Timer_100ms/1(TimerDebouncestatus) -> [RepeatTimer]
  Timer_800ms/2(Timer_Running_Status) -> [timer_running_status]
  [timer_800_status] -> Timer_100ms/2("ResetTimerStatus ")
  Data Store Read1/1 -> Timer_800ms/3(l_PrevTimerSt_In)
  Timer_800ms/3(l_PrevTimerSt_Out) -> Data Store Write1/1
  Timer_100ms/2(Timer_out) -> Data Store Write/1
  Data Store Read/1 -> Timer_100ms/3(Timer_In)
  AND/1 -> [l_RheDWLongPress_Tiout_sts], Logical Operator3/1
  Compare To Constant9/1 -> Logical Operator7/1
  [rheostatsw] -> Compare To Constant7/1
  [rheostatsw] -> Compare To Constant8/1, Compare To Constant9/1
  [timer_running_status] -> Logical Operator6/2
  [l_RheDWLongPress_sts] -> Logical Operator/1
  Logical Operator7/1 -> Logical Operator6/1
  Switch/1 -> " "/1
  Compare To Constant8/1 -> Logical Operator7/2
  [l_RheDWLongPress_Tiout_sts] -> Logical Operator/2
  Compare To Constant/1 -> AND/1
  [timer_800_status] -> Compare To Constant1/1, Unit Delay/1
  Unit Delay/1 -> Compare To Constant/1
  Logical Operator8/1 -> Switch/2
  Compare To Constant7/1 -> [l_RheDWLongPress_sts], Logical Operator5/1
  Compare To Constant1/1 -> AND/2
  [RepeatTimer] -> Logical Operator3/2
  Logical Operator5/1 -> Logical Operator8/1
  Constant2/1 -> Switch/1
  Constant5/1 -> Switch/3
  Logical Operator3/1 -> Logical Operator5/2
  Logical Operator6/1 -> [l_RheDWShortPress_sts], Logical Operator8/2
  Logical Operator/1 -> Enabled Subsystem/Enable
  [l_RheDWShortPress_sts] -> Enabled Subsystem1/Enable

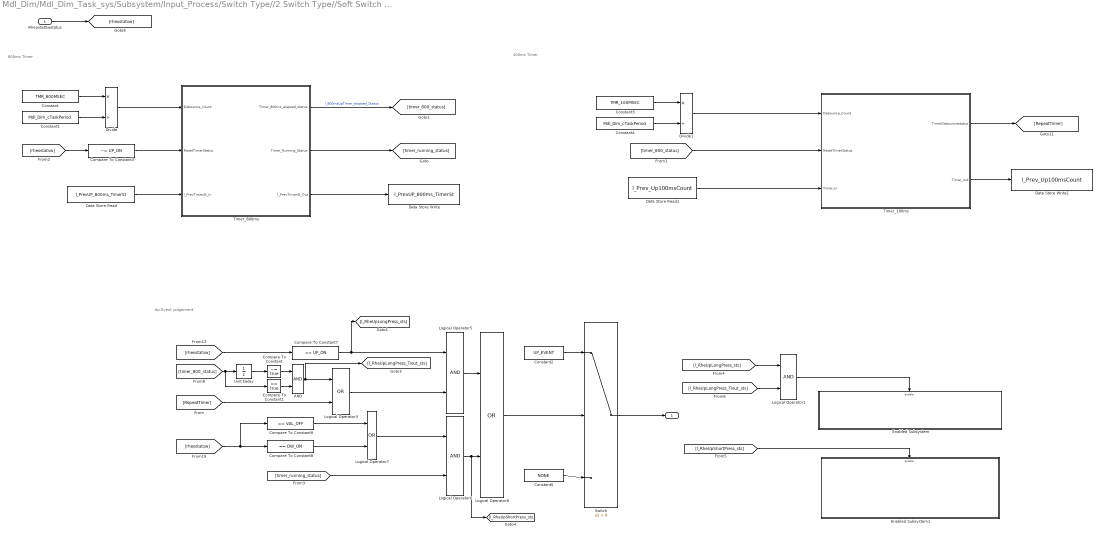
== system Mdl_Dim/Mdl_Dim_Task_sys/Subsystem/Input_Process/Switch Type//2 Switch Type//Soft Switch Type/RHEO_1SW_TYPE_AND_RHEO_2SW_TYPE/ Rheostat Up Event Determination ==
  note: 100ms Timer
  note: 800ms Timer
  note: Up Event judgement
  RheostatSwstatus : Inport
  AND : Logic  AllPortsSameDT=off  OutDataTypeStr=boolean
  Compare To Constant : simulink/Logic and Bit Operations/Compare To Constant  relop=~=  const=true  OutDataTypeStr=boolean
  Compare To Constant1 : simulink/Logic and Bit Operations/Compare To Constant  relop===  const=true  OutDataTypeStr=boolean
  Compare To Constant3 : simulink/Logic and Bit Operations/Compare To Constant  relop=~=  const=UP_ON  OutDataTypeStr=boolean
  Compare To Constant7 : simulink/Logic and Bit Operations/Compare To Constant  relop===  const=UP_ON  OutDataTypeStr=boolean
  Compare To Constant8 : simulink/Logic and Bit Operations/Compare To Constant  relop===  const=DW_ON  OutDataTypeStr=boolean
  Compare To Constant9 : simulink/Logic and Bit Operations/Compare To Constant  relop===  const=VAL_OFF  OutDataTypeStr=boolean
  Constant : Constant  Value=TMR_800MSEC
  Constant1 : Constant  Value=Mdl_Dim_cTaskPeriod
  Constant2 : Constant  Value=UP_EVENT
  Constant3 : Constant  Value=TMR_100MSEC
  Constant4 : Constant  Value=Mdl_Dim_cTaskPeriod
  Constant5 : Constant  Value=NONE
  Data Store Read : DataStoreRead  DataStoreName=l_PrevUP_800ms_TimerSt  IndexOptions=Index vector (dialog)  Indices=1  OutputSizes=1
  Data Store Read1 : DataStoreRead  DataStoreName=l_Prev_Up100msCount  IndexOptions=Index vector (dialog)  Indices=1  OutputSizes=1
  Data Store Write : DataStoreWrite  DataStoreName=l_PrevUP_800ms_TimerSt  IndexOptions=Index vector (dialog)  Indices=1  OutputSizes=1
  Data Store Write1 : DataStoreWrite  DataStoreName=l_Prev_Up100msCount  IndexOptions=Index vector (dialog)  Indices=1  OutputSizes=1
  Divide : Product  Inputs=*/  OutDataTypeStr=uint16
  Divide1 : Product  Inputs=*/  OutDataTypeStr=uint16
  Enabled Subsystem : Subsystem  TreatAsAtomicUnit=on
  Enabled Subsystem1 : Subsystem  TreatAsAtomicUnit=on
  Logical Operator1 : Logic  AllPortsSameDT=off  OutDataTypeStr=boolean
  Logical Operator3 : Logic  Operator=OR  AllPortsSameDT=off  OutDataTypeStr=boolean
  Logical Operator5 : Logic  AllPortsSameDT=off  OutDataTypeStr=boolean
  Logical Operator6 : Logic  AllPortsSameDT=off  OutDataTypeStr=boolean
  Logical Operator7 : Logic  Operator=OR  AllPortsSameDT=off  OutDataTypeStr=boolean
  Logical Operator8 : Logic  Operator=OR  AllPortsSameDT=off  OutDataTypeStr=boolean
  Switch : Switch  Criteria=u2 > Threshold  SaturateOnIntegerOverflow=off  InputSameDT=off
  Timer_100ms : Subsystem  Description=|  TreatAsAtomicUnit=on  RTWFcnName=Timer_100ms
      | Input 1 : Deboune Count
      | Input 2 : Reset Timer Status
      | Output : Timer Debounce Status
      settings: RTWFcnNameOpts=User specified
  Timer_800ms : Subsystem  Description=|  TreatAsAtomicUnit=on  RTWFcnName=Timer_800ms
      | Input 1 : Deboune Count
      | Input 2 : Reset Timer Status
      | Output : Timer Debounce Status
      settings: RTWFcnNameOpts=User specified
  Unit Delay : UnitDelay  SampleTime=-1  StateName=Prev_timer_800_status  HasFrameUpgradeWarning=on
  " " : Outport  VectorParamsAs1DForOutWhenUnconnected=off
  wires:
  Constant1/1 -> Divide/2
  Constant/1 -> Divide/1
  Timer_800ms/1(Timer_800ms_elapsed_status) -> [timer_800_status]  "l_800msUpTimer_elapsed_Status"
  Divide/1 -> Timer_800ms/1(Debounce_Count)
  Constant3/1 -> Divide1/1
  Constant4/1 -> Divide1/2
  RheostatSwstatus/1 -> [rheostatsw]
  [rheostatsw] -> Compare To Constant3/1
  Compare To Constant3/1 -> Timer_800ms/2("ResetTimerStatus ")
  Divide1/1 -> Timer_100ms/1(Debounce_Count)
  Timer_100ms/1(TimerDebouncestatus) -> [RepeatTimer]
  Timer_800ms/2(Timer_Running_Status) -> [timer_running_status]
  [timer_800_status] -> Timer_100ms/2("ResetTimerStatus ")
  Timer_800ms/3(l_PrevTimerSt_Out) -> Data Store Write/1
  Data Store Read/1 -> Timer_800ms/3(l_PrevTimerSt_In)
  Timer_100ms/2(Timer_out) -> Data Store Write1/1
  Data Store Read1/1 -> Timer_100ms/3(Timer_In)
  Switch/1 -> " "/1
  Logical Operator7/1 -> Logical Operator6/1
  [l_RheUpLongPress_Tiout_sts] -> Logical Operator1/2
  [l_RheUpLongPress_sts] -> Logical Operator1/1
  Unit Delay/1 -> Compare To Constant/1
  AND/1 -> [l_RheUpLongPress_Tiout_sts], Logical Operator3/1
  Logical Operator3/1 -> Logical Operator5/2
  [rheostatsw] -> Compare To Constant8/1, Compare To Constant9/1
  [timer_running_status] -> Logical Operator6/2
  Compare To Constant9/1 -> Logical Operator7/1
  [RepeatTimer] -> Logical Operator3/2
  [rheostatsw] -> Compare To Constant7/1
  Compare To Constant/1 -> AND/1
  Logical Operator5/1 -> Logical Operator8/1
  Logical Operator8/1 -> Switch/2
  Compare To Constant8/1 -> Logical Operator7/2
  Logical Operator6/1 -> [l_RheUpShortPress_sts], Logical Operator8/2
  Compare To Constant7/1 -> [l_RheUpLongPress_sts], Logical Operator5/1
  Compare To Constant1/1 -> AND/2
  Constant2/1 -> Switch/1
  [timer_800_status] -> Compare To Constant1/1, Unit Delay/1
  Constant5/1 -> Switch/3
  Logical Operator1/1 -> Enabled Subsystem/Enable
  [l_RheUpShortPress_sts] -> Enabled Subsystem1/Enable

== system Mdl_Dim/Mdl_Dim_Task_sys/Subsystem/Input_Process/Switch Type//2 Switch Type//Soft Switch Type/RHEO_1SW_TYPE_AND_RHEO_2SW_TYPE/50ms Timer ==
  RHUP_RawIn_Val : Inport
  AND : Logic  AllPortsSameDT=off  OutDataTypeStr=boolean
  Compare To Constant : simulink/Logic and Bit Operations/Compare To Constant  relop=~=  const=RHEO_VALUE_ZERO_BOOL  OutDataTypeStr=boolean
  Compare To Constant1 : simulink/Logic and Bit Operations/Compare To Constant  relop=~=  const=RHEO_VALUE_ONE_BOOL  OutDataTypeStr=boolean
  Compare To Constant5 : simulink/Logic and Bit Operations/Compare To Constant  relop===  const=RHEO_VALUE_ONE_BOOL  OutDataTypeStr=boolean
  Constant1 : Constant  Value=RHEO_VALUE_ZERO_U16  OutDataTypeStr=Inherit: Inherit via back propagation
  Constant4 : Constant  Value=RHEO_VALUE_ONE_U16  OutDataTypeStr=uint16
  Constant5 : Constant  Value=RHEO_VALUE_ZERO_U16  OutDataTypeStr=Inherit: Inherit via back propagation
  Constant7 : Constant  Value=RHEO_VALUE_FIVE_U16  OutDataTypeStr=uint16
  Subtract1 : Sum  Inputs=+-
  Switch2 : Switch  Criteria=u2 ~= 0  OutDataTypeStr=uint16  SaturateOnIntegerOverflow=off  InputSameDT=off
  Switch3 : Switch  Criteria=u2 ~= 0  OutDataTypeStr=uint16  RndMeth=Simplest  SaturateOnIntegerOverflow=off  InputSameDT=off
  Unit Delay : UnitDelay  SampleTime=-1  StateName=Prev_RHUP_RawIn_Val  HasFrameUpgradeWarning=on
  Unit Delay2 : UnitDelay  InitialCondition=ZERO_DUTY  SampleTime=-1  StateName=Prev_SW1Rheostat_Up_time_Step50ms  HasFrameUpgradeWarning=on
  check count2 : RelationalOperator  Operator=~=  OutDataTypeStr=boolean  InputSameDT=off
  RHUP_RawIn_Val_50ms : Outport  VectorParamsAs1DForOutWhenUnconnected=off
  wires:
  Unit Delay2/1 -> Switch2/3  "current_count_2"
  Switch2/1 -> Subtract1/1, check count2/1  "current_count_2"
  check count2/1 -> RHUP_RawIn_Val_50ms/1, Switch3/2  "fl_RHUP_RawIn_Val_50ms"
  Compare To Constant5/1 -> Switch2/2
  Constant4/1 -> Subtract1/2  "Decrement_Value_2"
  Constant7/1 -> Switch2/1  "Decrement_Value_2fRheo"
  Switch3/1 -> Unit Delay2/1
  Constant5/1 -> check count2/2  "Max_step_Count2"
  RHUP_RawIn_Val/1 -> [RHUP_RawIn_Val], Unit Delay/1
  Unit Delay/1 -> [Prev_RHUP_RawIn_Val]
  AND/1 -> Compare To Constant5/1
  Subtract1/1 -> Switch3/1  "current_count_2"
  Constant1/1 -> Switch3/3
  [RHUP_RawIn_Val] -> Compare To Constant/1
  Compare To Constant/1 -> AND/1
  Compare To Constant1/1 -> AND/2
  [Prev_RHUP_RawIn_Val] -> Compare To Constant1/1

== system Mdl_Dim/Mdl_Dim_Task_sys/Subsystem/Input_Process/Switch Type//2 Switch Type//Soft Switch Type/RHEO_1SW_TYPE_AND_RHEO_2SW_TYPE/If Action Subsystem1 ==
  Action Port : ActionPort
  Constant : Constant  Value=VAL_ON  OutDataTypeStr=uint8
  RHUP_Dbc_Status : Outport  VectorParamsAs1DForOutWhenUnconnected=off
  wires:
  Constant/1 -> RHUP_Dbc_Status/1

== system Mdl_Dim/Mdl_Dim_Task_sys/Subsystem/Input_Process/Switch Type//2 Switch Type//Soft Switch Type/RHEO_1SW_TYPE_AND_RHEO_2SW_TYPE/If Action Subsystem10 ==
  In1 : Inport
  Action Port : ActionPort
  RHDW_Dbc_Status : Outport  VectorParamsAs1DForOutWhenUnconnected=off
  wires:
  In1/1 -> RHDW_Dbc_Status/1

== system Mdl_Dim/Mdl_Dim_Task_sys/Subsystem/Input_Process/Switch Type//2 Switch Type//Soft Switch Type/RHEO_1SW_TYPE_AND_RHEO_2SW_TYPE/If Action Subsystem2 ==
  Action Port : ActionPort
  Constant : Constant  Value=VAL_ON  OutDataTypeStr=uint8
  RHUP_Dbc_Status : Outport  VectorParamsAs1DForOutWhenUnconnected=off
  wires:
  Constant/1 -> RHUP_Dbc_Status/1

== system Mdl_Dim/Mdl_Dim_Task_sys/Subsystem/Input_Process/Switch Type//2 Switch Type//Soft Switch Type/RHEO_1SW_TYPE_AND_RHEO_2SW_TYPE/If Action Subsystem3 ==
  Action Port : ActionPort
  Constant : Constant  Value=VAL_OFF  OutDataTypeStr=uint8
  RHUP_Dbc_Status : Outport  VectorParamsAs1DForOutWhenUnconnected=off
  wires:
  Constant/1 -> RHUP_Dbc_Status/1

== system Mdl_Dim/Mdl_Dim_Task_sys/Subsystem/Input_Process/Switch Type//2 Switch Type//Soft Switch Type/RHEO_1SW_TYPE_AND_RHEO_2SW_TYPE/If Action Subsystem4 ==
  Action Port : ActionPort
  Constant : Constant  Value=VAL_OFF  OutDataTypeStr=uint8
  RHUP_Dbc_Status : Outport  VectorParamsAs1DForOutWhenUnconnected=off
  wires:
  Constant/1 -> RHUP_Dbc_Status/1

== system Mdl_Dim/Mdl_Dim_Task_sys/Subsystem/Input_Process/Switch Type//2 Switch Type//Soft Switch Type/RHEO_1SW_TYPE_AND_RHEO_2SW_TYPE/If Action Subsystem5 ==
  In1 : Inport
  Action Port : ActionPort
  RHUP_Dbc_Status : Outport  VectorParamsAs1DForOutWhenUnconnected=off
  wires:
  In1/1 -> RHUP_Dbc_Status/1

== system Mdl_Dim/Mdl_Dim_Task_sys/Subsystem/Input_Process/Switch Type//2 Switch Type//Soft Switch Type/RHEO_1SW_TYPE_AND_RHEO_2SW_TYPE/If Action Subsystem6 ==
  Action Port : ActionPort
  Constant : Constant  Value=VAL_ON  OutDataTypeStr=uint8
  RHDW_Dbc_Status : Outport  VectorParamsAs1DForOutWhenUnconnected=off
  wires:
  Constant/1 -> RHDW_Dbc_Status/1

== system Mdl_Dim/Mdl_Dim_Task_sys/Subsystem/Input_Process/Switch Type//2 Switch Type//Soft Switch Type/RHEO_1SW_TYPE_AND_RHEO_2SW_TYPE/If Action Subsystem7 ==
  Action Port : ActionPort
  Constant : Constant  Value=VAL_ON  OutDataTypeStr=uint8
  RHDW_Dbc_Status : Outport  VectorParamsAs1DForOutWhenUnconnected=off
  wires:
  Constant/1 -> RHDW_Dbc_Status/1

== system Mdl_Dim/Mdl_Dim_Task_sys/Subsystem/Input_Process/Switch Type//2 Switch Type//Soft Switch Type/RHEO_1SW_TYPE_AND_RHEO_2SW_TYPE/If Action Subsystem8 ==
  Action Port : ActionPort
  Constant : Constant  Value=VAL_OFF  OutDataTypeStr=uint8
  RHDW_Dbc_Status : Outport  VectorParamsAs1DForOutWhenUnconnected=off
  wires:
  Constant/1 -> RHDW_Dbc_Status/1

== system Mdl_Dim/Mdl_Dim_Task_sys/Subsystem/Input_Process/Switch Type//2 Switch Type//Soft Switch Type/RHEO_1SW_TYPE_AND_RHEO_2SW_TYPE/If Action Subsystem9 ==
  Action Port : ActionPort
  Constant : Constant  Value=VAL_OFF  OutDataTypeStr=uint8
  RHDW_Dbc_Status : Outport  VectorParamsAs1DForOutWhenUnconnected=off
  wires:
  Constant/1 -> RHDW_Dbc_Status/1

== system Mdl_Dim/Mdl_Dim_Task_sys/Subsystem/Input_Process/Switch Type//2 Switch Type//Soft Switch Type/RHEO_1SW_TYPE_AND_RHEO_2SW_TYPE/Rheostat_ONS_Status_Output  ==
  Trigger_Event : Inport
  AND : Logic  AllPortsSameDT=off  OutDataTypeStr=boolean
  AND1 : Logic  AllPortsSameDT=off  OutDataTypeStr=boolean
  Compare To Constant : simulink/Logic and Bit Operations/Compare To Constant  relop===  const=VAL_ZERO  OutDataTypeStr=boolean
  Compare To Constant7 : simulink/Logic and Bit Operations/Compare To Constant  relop===  const=VAL_ONE  OutDataTypeStr=boolean
  Compare To Constant8 : simulink/Logic and Bit Operations/Compare To Constant  relop===  const=VAL_TWO  OutDataTypeStr=boolean
  Constant3 : Constant  Value=TMR_3000MSEC
  Constant4 : Constant  Value=Mdl_Dim_cTaskPeriod
  Data Store Read1 : DataStoreRead  DataStoreName=RheostatONSStatus  IndexOptions=Index vector (dialog)  Indices=1  OutputSizes=1
  Data Store Read2 : DataStoreRead  DataStoreName=RheostatONSStatus  IndexOptions=Index vector (dialog)  Indices=1  OutputSizes=1
  Data Store Read3 : DataStoreRead  DataStoreName=RheostatONSStatus  IndexOptions=Index vector (dialog)  Indices=1  OutputSizes=1
  Debounce_timer_Subsystem2 : Subsystem  Description=|
      | Input 1 : Deboune Count
      | Input 2 : Reset Timer Status
      | Output : Timer Debounce Status
  Divide1 : Product  Inputs=*/  OutDataTypeStr=uint16
  If3 : If  NumInputs=2  IfExpression=(u1 ~= 0)  ElseIfExpressions=(u2 ~= 0)
  OR : Logic  Operator=OR  AllPortsSameDT=off  OutDataTypeStr=boolean
  Subsystem3 : Subsystem
  Subsystem4 : Subsystem
  Subsystem5 : Subsystem
  pp_RheostatONSStatus_RheostatONSStatus_In : Outport  VectorParamsAs1DForOutWhenUnconnected=off
  wires:
  [Trigger_Event] -> AND1/2
  If3/3 -> Subsystem5/Action
  If3/2 -> Subsystem4/Action
  Constant3/1 -> Divide1/1
  Data Store Read1/1 -> Compare To Constant/1, Compare To Constant8/1
  Data Store Read3/1 -> Compare To Constant7/1
  [Temp_ON2] -> If3/2
  [Temp_ON1] -> If3/1
  AND1/1 -> [Temp_ON2]
  Data Store Read2/1 -> pp_RheostatONSStatus_RheostatONSStatus_In/1
  If3/1 -> Subsystem3/Action
  Compare To Constant/1 -> OR/1
  Compare To Constant7/1 -> AND1/1
  Compare To Constant8/1 -> OR/2
  Constant4/1 -> Divide1/2
  Divide1/1 -> Debounce_timer_Subsystem2/1(Debounce_Count)
  OR/1 -> AND/1
  [Trigger_Event] -> AND/2
  AND/1 -> [Temp_ON1]
  [Trigger_Event] -> Debounce_timer_Subsystem2/2("ResetTimerStatus ")
  Trigger_Event/1 -> [Trigger_Event]

== system Mdl_Dim/Mdl_Dim_Task_sys/Subsystem/Input_Process/Switch Type//2 Switch Type//Soft Switch Type/RHEO_1SW_TYPE_AND_RHEO_2SW_TYPE/Subsystem ==
  RHEO_SW_IN_ADIN_Val : Inport
  Action Port : ActionPort
  Truth Table : Truth Table  TreatAsAtomicUnit=on
  RHUP_RawIn_Val : Outport  VectorParamsAs1DForOutWhenUnconnected=off
  ADC_RHDW_val : Outport  Port=2  VectorParamsAs1DForOutWhenUnconnected=off
  wires:
  RHEO_SW_IN_ADIN_Val/1 -> Truth Table/1(RHEO_SW_IN_ADIN_Val)
  Truth Table/2(RHDW_RawIn_Val) -> ADC_RHDW_val/1
  Truth Table/1(RHUP_RawIn_Val) -> RHUP_RawIn_Val/1

== system Mdl_Dim/Mdl_Dim_Task_sys/Subsystem/Input_Process/Switch Type//2 Switch Type//Soft Switch Type/RHEO_1SW_TYPE_AND_RHEO_2SW_TYPE/Subsystem1 ==
  RHEO_SW_IN_ADIN_Val : Inport
  RHEO_SW_DOWN : Inport  Port=2
  Action Port : ActionPort
  Cast : DataTypeConversion  OutDataTypeStr=boolean  SaturateOnIntegerOverflow=off  RndMeth=Floor
  Compare To Constant2 : simulink/Logic and Bit Operations/Compare To Constant  relop=<  const=UP_THRESH_2SW  OutDataTypeStr=boolean
  Constant2 : Constant  Value=true
  Constant3 : Constant  Value=false
  Switch : Switch  Criteria=u2 ~= 0  SaturateOnIntegerOverflow=off  InputSameDT=off
  RHUP_RawIn_Val : Outport  VectorParamsAs1DForOutWhenUnconnected=off
  ADC_RHDW_val : Outport  Port=2  VectorParamsAs1DForOutWhenUnconnected=off
  wires:
  RHEO_SW_IN_ADIN_Val/1 -> Compare To Constant2/1
  RHEO_SW_DOWN/1 -> Cast/1
  Switch/1 -> RHUP_RawIn_Val/1
  Compare To Constant2/1 -> Switch/2
  Constant2/1 -> Switch/1
  Constant3/1 -> Switch/3
  Cast/1 -> ADC_RHDW_val/1
